simulink subsystem "F16_Quaternion"  (R2023b)
settings: Solver=VariableStepAuto  StartTime=0.0  StopTime=10.0  RelTol=1e-3
undefined symbols (not defined in the file): controlDeflections, dataBase, deltaLEF, e0_0, e1_0, e2_0, e3_0, pm_0, statesFinal, Vm_0, xme_0
libraries: sharedtransform x4, aerolibtransform2 x2, matrix_library x2, shared6dof x1
(part 1 of 2)
settings Model: Creator=cyber  LastModifiedBy=cyber

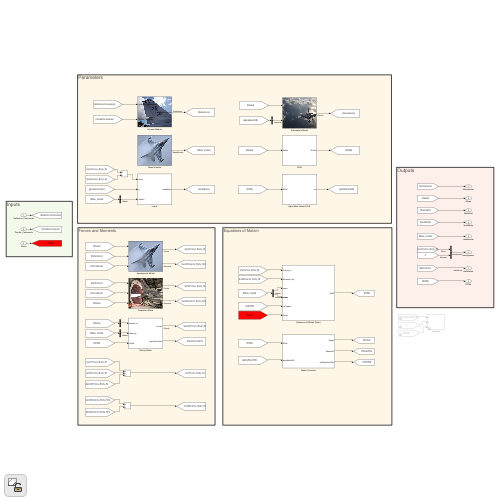
[thumbnail: Simulink's stored preview of the top-level diagram]
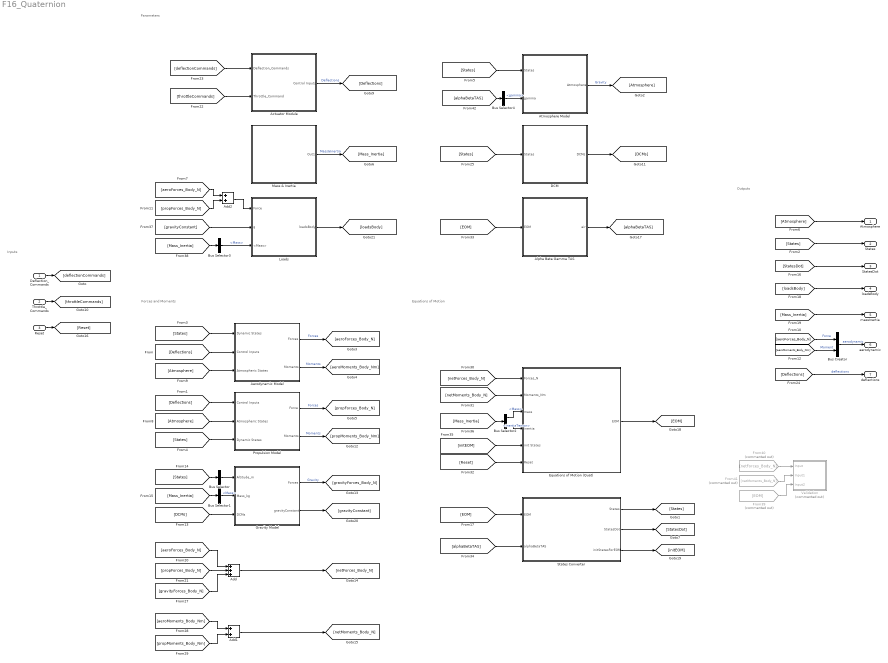
== system F16_Quaternion ==
  note: Forces and Moments
  note: Outputs
  note: Inputs
  note: Parameters
  note: Equations of Motion
  Deflection_Commands : Inport
  Throttle_Commands : Inport  Port=2
  Reset : Inport  Port=3
  Actuator Module : Subsystem
      mask Display: image('F16_ControlSurface.png'); % Use "Edit Image" on toolstrip to change.
  Add : Sum  Inputs=+++
  Add1 : Sum
  Add2 : Sum
  Aerodynamic Model : Subsystem
      mask Display: image('F16.PNG'); % Use "Edit Image" on toolstrip to change.
  "Alpha Beta Gamma TAS " : Subsystem
  Atmosphere Model : Subsystem
      mask Display: image('f16_atm.jpg'); % Use "Edit Image" on toolstrip to change.
  Bus Creator : BusCreator  Inputs=2
  Bus Selector : BusSelector  OutputSignals=Altitude  OutputAsBus=on
  Bus Selector1 : BusSelector  OutputSignals=Mass
  Bus Selector2 : BusSelector  OutputSignals=Mass,inertiaTensor
  Bus Selector3 : BusSelector  OutputSignals=Mass
  Bus Selector4 : BusSelector  OutputSignals=gamma
  DCM : Subsystem
  Equations of Motion (Quat) : Subsystem
  From39 : From  Commented=on  GotoTag=EOM
  From40 : From  Commented=on  GotoTag=netForces_Body_N
  From41 : From  Commented=on  GotoTag=netMoments_Body_N
  "Gravity Model " : Subsystem
  Loads : Subsystem
  Mass & Inertia : Subsystem
      mask Display: image('F16.PNG'); % Use "Edit Image" on toolstrip to change.
  Propulsion Model : Subsystem
      mask Display: image('F16_Engine.PNG'); % Use "Edit Image" on toolstrip to change.
  States Converter : Subsystem
  Validation : Subsystem  Commented=on
  Atmosphere : Outport
  States : Outport  Port=2
  StatesDot : Outport  Port=3
  loadsBody : Outport  Port=4
  massInertia : Outport  Port=5
  aerodynamic : Outport  Port=6
  deflections : Outport  Port=7
  wires:
  DCM/1(DCMs) -> [DCMs]
  [States] -> DCM/1(States)
  [Deflections] -> deflections/1  "deflections"
  Throttle_Commands/1 -> [throttleCommands]
  [deflectionCommands] -> Actuator Module/1(Deflection_Commands)
  Actuator Module/1(Control Inputs) -> [Deflections]  "Deflections"
  [throttleCommands] -> Actuator Module/2(Throttle_Command)
  Bus Creator/1 -> aerodynamic/1  "aerodynamic"
  [aeroMoments_Body_Nm] -> Bus Creator/2  "Moment"
  [aeroForces_Body_N] -> Bus Creator/1  "Force"
  [Mass_Inertia] -> massInertia/1
  [loadsBody] -> loadsBody/1
  [StatesDot] -> StatesDot/1
  [Atmosphere] -> Aerodynamic Model/3(Atmospheric States)
  [Atmosphere] -> Propulsion Model/2(Atmospheric States)
  [Atmosphere] -> Atmosphere/1
  [States] -> Atmosphere Model/1(States)
  [States] -> Propulsion Model/3(Dynamic States)
  [States] -> Aerodynamic Model/1(Dynamic States)
  [States] -> States/1
  [Deflections] -> Propulsion Model/1(Control Inputs)
  Deflection_Commands/1 -> [deflectionCommands]
  States Converter/2(StatesDot) -> [StatesDot]
  Atmosphere Model/1(Atmosphere) -> [Atmosphere]  "Gravity"
  [Deflections] -> Aerodynamic Model/2(Control Inputs)
  Aerodynamic Model/1(Forces) -> [aeroForces_Body_N]  "Forces"
  Aerodynamic Model/2(Moments) -> [aeroMoments_Body_Nm]  "Moments"
  States Converter/1(States) -> [States]
  Mass & Inertia/1(Out1) -> [Mass_Inertia]  "Mass&Inertia"
  Propulsion Model/2(Moments) -> [propMoments_Body_Nm]  "Moments"
  Propulsion Model/1(Force) -> [propForces_Body_N]  "Forces"
  [DCMs] -> "Gravity Model "/3(DCMs)
  [States] -> Bus Selector/1
  Bus Selector/1 -> "Gravity Model "/1(Altitude_m)
  [Mass_Inertia] -> Bus Selector1/1
  Bus Selector1/1 -> "Gravity Model "/2(Mass_kg)  "<Mass>"
  "Gravity Model "/1(Forces) -> [gravityForces_Body_N]  "Gravity"
  [propForces_Body_N] -> Add/2
  [aeroForces_Body_N] -> Add/1
  [gravityForces_Body_N] -> Add/3
  Add/1 -> [netForces_Body_N]
  [aeroMoments_Body_Nm] -> Add1/1
  [propMoments_Body_Nm] -> Add1/2
  Add1/1 -> [netMoments_Body_N]
  [netForces_Body_N] -> Equations of Motion (Quat)/1(Forces_N)
  [netMoments_Body_N] -> Equations of Motion (Quat)/2(Moments_Nm)
  Reset/1 -> [Reset]
  [Reset] -> Equations of Motion (Quat)/6(Reset)
  "Alpha Beta Gamma TAS "/1(air) -> [alphaBetaTAS]
  Equations of Motion (Quat)/1(EOM) -> [EOM]
  [EOM] -> "Alpha Beta Gamma TAS "/1(EOM)
  [EOM] -> States Converter/1(EOM)
  [alphaBetaTAS] -> States Converter/2(alphaBetaTAS)
  States Converter/3(initStatesForEOM) -> [initEOM]
  [initEOM] -> Equations of Motion (Quat)/5(init States)
  [Mass_Inertia] -> Bus Selector2/1
  Bus Selector2/1 -> Equations of Motion (Quat)/3(mass)  "<Mass>"
  Bus Selector2/2 -> Equations of Motion (Quat)/4(inertia)  "<inertiaTensor>"
  "Gravity Model "/2(gravityConstant) -> [gravityConstant]
  Bus Selector3/1 -> Loads/3(<Mass>)  "<Mass>"
  [aeroForces_Body_N] -> Add2/1
  [propForces_Body_N] -> Add2/2
  Add2/1 -> Loads/1(Force)
  [gravityConstant] -> Loads/2(g)
  [Mass_Inertia] -> Bus Selector3/1
  Loads/1(loadsBody) -> [loadsBody]
  From39/1 -> Validation/3(Input2)
  From41/1 -> Validation/2(Input1)
  From40/1 -> Validation/1(Input)
  [alphaBetaTAS] -> Bus Selector4/1
  Bus Selector4/1 -> Atmosphere Model/2(gamma)  "<gamma>"

== system F16_Quaternion/Actuator Module ==
  Deflection_Commands : Inport
  Throttle_Command : Inport  Port=2
  Bus Creator : BusCreator  Inputs=6
  Demux : Demux  Outputs=6
  First Order Aileron Actuator : Subsystem
  First Order HT Actuator : Subsystem
  First Order Rudder Actuator : Subsystem
  First Order Throttle Actuator : Subsystem
  Leading Edge Flap : Constant  Value=deltaLEF
  Speed Brake : Constant  Value=0
  Terminator : Terminator
  Terminator1 : Terminator
  Terminator2 : Terminator
  Control Inputs : Outport
  wires:
  Bus Creator/1 -> Control Inputs/1
  First Order Throttle Actuator/1(Output) -> Bus Creator/4  "Throttle"
  Speed Brake/1 -> Bus Creator/6  "Speed Brake"
  Demux/1 -> [HorizontalTail]
  Demux/2 -> [Aileron]
  Demux/3 -> [Rudder]
  Demux/4 -> Terminator/1
  Demux/5 -> Terminator2/1
  Demux/6 -> Terminator1/1
  Deflection_Commands/1 -> Demux/1
  Leading Edge Flap/1 -> Bus Creator/5  "LEF"
  [HorizontalTail] -> First Order HT Actuator/1(Deflection)  "Horizontal Tail Command"
  [Aileron] -> First Order Aileron Actuator/1(Deflection)  "Aileron Command"
  [Rudder] -> First Order Rudder Actuator/1(Deflection)  "Rudder Command"
  First Order HT Actuator/1(Output) -> Bus Creator/1  "Horizontal Tail"
  First Order Aileron Actuator/1(Output) -> Bus Creator/2  "Aileron"
  First Order Rudder Actuator/1(Output) -> Bus Creator/3  "Rudder"
  Throttle_Command/1 -> [Throttle_Command]
  [Throttle_Command] -> First Order Throttle Actuator/1(Deflection)  "Throttle Command"

== system F16_Quaternion/Aerodynamic Model ==
  Dynamic States : Inport
  Control Inputs : Inport  Port=2
  Atmospheric States : Inport  Port=3
  Bus Creator : BusCreator  Inputs=2
  Bus Selector : BusSelector  OutputSignals=Dynamic Pressure
  Constant : Constant  Value=dataBase.Sw
  Demux1 : Demux  Outputs=3
  Force Coeffs : Subsystem
  Gain : Gain  Gain=dataBase.MAC*dataBase.Sw
  Gain1 : Gain  Gain=dataBase.b*dataBase.Sw
  Gain2 : Gain  Gain=dataBase.b*dataBase.Sw
  Moment Coeffs : Subsystem
  Mux : Mux  Inputs=3
  Mux1 : Mux  Inputs=3
  Mux2 : Mux  Inputs=3
  Product : Product  Inputs=3
  Product1 : Product
  Product2 : Product
  Product3 : Product
  Selector : Selector  InputPortWidth=3  IndexOptions=Index vector (dialog)  Indices=[2,1,3]  OutputSizes=1
  Forces : Outport
  Moments : Outport  Port=2
  wires:
  Selector/1 -> Moments/1
  Force Coeffs/3(" CZ") -> Bus Creator/2, Mux/3  "CZ"
  Force Coeffs/2(" CY") -> Bus Creator/1, Mux/2  "CY"
  Force Coeffs/1(" CX") -> Mux/1
  Mux/1 -> Product/2
  Moment Coeffs/1(" Cm") -> Mux1/1
  Mux1/1 -> Demux1/1
  Moment Coeffs/3(" Cn") -> Mux1/3
  Moment Coeffs/2(" Cl") -> Mux1/2
  Bus Creator/1 -> Moment Coeffs/1(Force Effects on Moments)
  Dynamic States/1 -> Moment Coeffs/2(Dynamic States), Force Coeffs/1(Dynamic States)
  Control Inputs/1 -> Moment Coeffs/3(Control Inputs), Force Coeffs/2(Control Inputs)
  Atmospheric States/1 -> Bus Selector/1
  Bus Selector/1 -> [DynamicPressure]  "<Dynamic Pressure>"
  [DynamicPressure] -> Product/1
  Constant/1 -> Product/3
  Product/1 -> Forces/1
  Demux1/1 -> Gain/1
  Gain/1 -> Product1/2
  [DynamicPressure] -> Product2/1, Product3/1, Product1/1
  Demux1/2 -> Gain1/1
  Demux1/3 -> Gain2/1
  Gain1/1 -> Product2/2
  Gain2/1 -> Product3/2
  Product3/1 -> Mux2/3
  Product2/1 -> Mux2/2
  Product1/1 -> Mux2/1
  Mux2/1 -> Selector/1

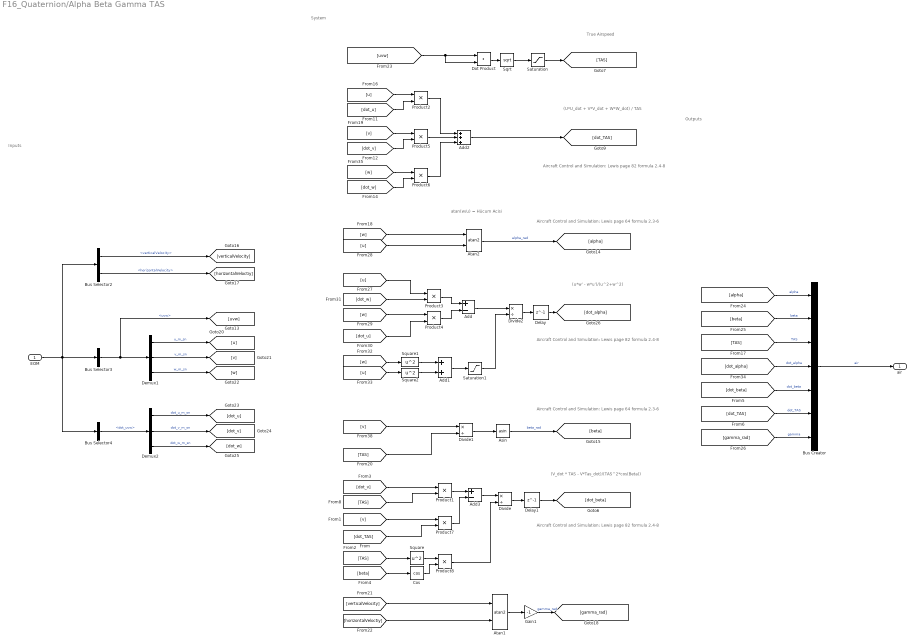
== system F16_Quaternion/Alpha Beta Gamma TAS  ==
  note: Aircraft Control and Simulation: Lewis page 64 formula 2.3-6
  note: Aircraft Control and Simulation: Lewis page 64 formula 2.3-6
  note: Aircraft Control and Simulation: Lewis page 82 formula 2.4-8
  note: Aircraft Control and Simulation: Lewis page 82 formula 2.4-8
  note: System
  note: Outputs
  note: Inputs
  note: (u*w' - w*u')/(u^2+w^2)
  note: atan(w/u) = Hücum Acisi
  note: Aircraft Control and Simulation: Lewis page 82 formula 2.4-8
  note: (U*U_dot + V*V_dot + W*W_dot) / TAS
  note: (V_dot * TAS - V*Tas_dot)/(TAS^2*cos(Beta))
  note: True Airspeed
  EOM : Inport  OutDataTypeStr=double
  Add : Sum  Inputs=+-
  Add1 : Sum
  Add2 : Sum  Inputs=3
  Add3 : Sum  Inputs=+-
  Asin : Trigonometry  Operator=asin
  Atan1 : Trigonometry  Operator=atan2
  Atan2 : Trigonometry  Operator=atan2
  Bus Creator : BusCreator  Inputs=7
  Bus Selector2 : BusSelector  OutputSignals=verticalVelocity,horizontalVelocity
  Bus Selector3 : BusSelector  OutputSignals=uvw
  Bus Selector4 : BusSelector  OutputSignals=dot_uvw
  Cos : Trigonometry  Operator=cos
  Delay : Delay  DelayLength=1  InitialCondition=0
  Delay1 : Delay  DelayLength=1
  Demux1 : Demux  Outputs=3
  Demux2 : Demux  Outputs=3
  Divide : Product  Inputs=*/
  Divide1 : Product  Inputs=*/
  Divide2 : Product  Inputs=*/
  Dot Product : DotProduct  OutDataTypeStr=Inherit: Inherit via internal rule
  Gain1 : Gain  Gain=-1
  Product{1..8} (8 alike) : Product
  Saturation : Saturate  UpperLimit=inf  LowerLimit=0.000000001
  Saturation1 : Saturate  UpperLimit=inf  LowerLimit=0.000000001
  Sqrt : Sqrt
  Square : Math  Operator=square
  Square1 : Math  Operator=square
  Square2 : Math  Operator=square
  air : Outport
  wires:
  [gamma_rad] -> Bus Creator/7  "gamma"
  [dot_TAS] -> Bus Creator/6  "dot_TAS"
  [dot_beta] -> Bus Creator/5  "dot_beta"
  [dot_alpha] -> Bus Creator/4  "dot_alpha"
  [alpha] -> Bus Creator/1  "alpha"
  [TAS] -> Bus Creator/3  "TAS"
  [beta] -> Bus Creator/2  "beta"
  Divide/1 -> Delay1/1
  Product8/1 -> Divide/2
  Cos/1 -> Product8/2
  Square/1 -> Product8/1
  [beta] -> Cos/1
  Add3/1 -> Divide/1
  [TAS] -> Square/1
  [v] -> Product7/1
  [dot_TAS] -> Product7/2
  Product7/1 -> Add3/2
  Product1/1 -> Add3/1
  [TAS] -> Product1/2
  [dot_v] -> Product1/1
  Delay1/1 -> [dot_beta]
  Add2/1 -> [dot_TAS]
  Product2/1 -> Add2/1
  Product6/1 -> Add2/3
  Product5/1 -> Add2/2
  [dot_w] -> Product6/2
  [w] -> Product6/1
  [v] -> Product5/1
  [dot_v] -> Product5/2
  [dot_u] -> Product2/2
  [u] -> Product2/1
  Delay/1 -> [dot_alpha]
  Saturation1/1 -> Divide2/2
  Saturation/1 -> [TAS]
  Divide2/1 -> Delay/1
  Add1/1 -> Saturation1/1
  Square2/1 -> Add1/2
  Square1/1 -> Add1/1
  [u] -> Square2/1
  [w] -> Square1/1
  Add/1 -> Divide2/1
  Product4/1 -> Add/2
  Product3/1 -> Add/1
  [dot_u] -> Product4/2
  [w] -> Product4/1
  [dot_w] -> Product3/2
  [u] -> Product3/1
  Bus Selector4/1 -> Demux2/1  "<dot_uvw>"
  Demux2/1 -> [dot_u]  "dot_u_m_sn"
  Demux2/2 -> [dot_v]  "dot_v_m_sn"
  Demux2/3 -> [dot_w]  "dot_w_m_sn"
  Demux1/3 -> [w]  "w_m_sn"
  Demux1/2 -> [v]  "v_m_sn"
  Demux1/1 -> [u]  "u_m_sn"
  [uvw] -> Dot Product/1, Dot Product/2
  Sqrt/1 -> Saturation/1
  Dot Product/1 -> Sqrt/1
  Gain1/1 -> [gamma_rad]  "gamma_rad"
  Atan1/1 -> Gain1/1
  [horizontalVeloctiy] -> Atan1/2
  [verticalVelocity] -> Atan1/1
  Bus Selector2/2 -> [horizontalVeloctiy]  "<horizontalVelocity>"
  Bus Selector2/1 -> [verticalVelocity]  "<verticalVelocity>"
  Asin/1 -> [beta]  "beta_rad"
  Divide1/1 -> Asin/1
  [TAS] -> Divide1/2
  [v] -> Divide1/1
  Atan2/1 -> [alpha]  "alpha_rad"
  [w] -> Atan2/1
  [u] -> Atan2/2
  Bus Selector3/1 -> Demux1/1, [uvw]  "<uvw>"
  EOM/1 -> Bus Selector3/1, Bus Selector2/1, Bus Selector4/1
  Bus Creator/1 -> air/1  "air"

== system F16_Quaternion/Atmosphere Model ==
  States : Inport
  gamma : Inport  Port=2
  Bus Creator : BusCreator  Inputs=8
  Bus Selector : BusSelector  OutputSignals=Altitude,Velocity
  MATLAB Function : MATLAB Function  TreatAsAtomicUnit=on
  Atmosphere : Outport
  wires:
  MATLAB Function/7(speedOfSound) -> Bus Creator/7  "speedOfSound"
  gamma/1 -> Bus Creator/8  "gamma"
  States/1 -> Bus Selector/1
  MATLAB Function/2(T) -> Bus Creator/2  "Temperature"
  MATLAB Function/3(P) -> Bus Creator/3  "Pressure"
  MATLAB Function/4(rho) -> Bus Creator/4  "Density"
  MATLAB Function/5(Qdyn) -> Bus Creator/5  "Dynamic Pressure"
  MATLAB Function/6(M) -> Bus Creator/6  "Mach"
  MATLAB Function/1(g) -> Bus Creator/1  "Gravity"
  Bus Creator/1 -> Atmosphere/1
  Bus Selector/1 -> MATLAB Function/1(h)  "<Altitude>"
  Bus Selector/2 -> MATLAB Function/2(V)  "<Velocity>"

== system F16_Quaternion/DCM ==
  note: Body to Wind
  note: Body to Stability
  note: Earth to Body
  States : Inport
  Bus Creator : BusCreator  Inputs=3
  Bus Selector : BusSelector  OutputSignals=Phi,Theta,Psi,Alpha,Beta
  Constant1 : Constant  Value=0
  Direction Cosine Matrix Body to Wind1 : aerolibtransform2/Direction Cosine Matrix Body to Wind
  Direction Cosine Matrix Body to Wind2 : aerolibtransform2/Direction Cosine Matrix Body to Wind
  Mux : Mux  Inputs=3
  Mux1 : Mux  Inputs=2
  Mux3 : Mux  Inputs=2
  Rotation Angles to Direction Cosine Matrix : sharedtransform/Rotation Angles to Direction Cosine Matrix  rotationOrder=ZYX  aMode=aMode
  DCMs : Outport
  wires:
  Bus Selector/5 -> [beta]  "<Beta>"
  [beta] -> Mux1/2  "beta_rad"
  Mux1/1 -> Direction Cosine Matrix Body to Wind2/1
  [alpha] -> Mux1/1
  Direction Cosine Matrix Body to Wind2/1 -> Bus Creator/3  "DCMwb"
  Bus Selector/4 -> [alpha]  "<Alpha>"
  Direction Cosine Matrix Body to Wind1/1 -> Bus Creator/2  "DCMsb"
  [alpha] -> Mux3/1
  Mux3/1 -> Direction Cosine Matrix Body to Wind1/1
  Constant1/1 -> Mux3/2  "beta_rad"
  Mux/1 -> Rotation Angles to Direction Cosine Matrix/1
  States/1 -> Bus Selector/1
  Bus Selector/1 -> [phi]  "<Phi>"
  Bus Selector/2 -> [theta]  "<Theta>"
  Bus Selector/3 -> [psi]  "<Psi>"
  [theta] -> Mux/2
  [phi] -> Mux/3
  [psi] -> Mux/1
  Rotation Angles to Direction Cosine Matrix/1 -> Bus Creator/1  "DCMbe"
  Bus Creator/1 -> DCMs/1

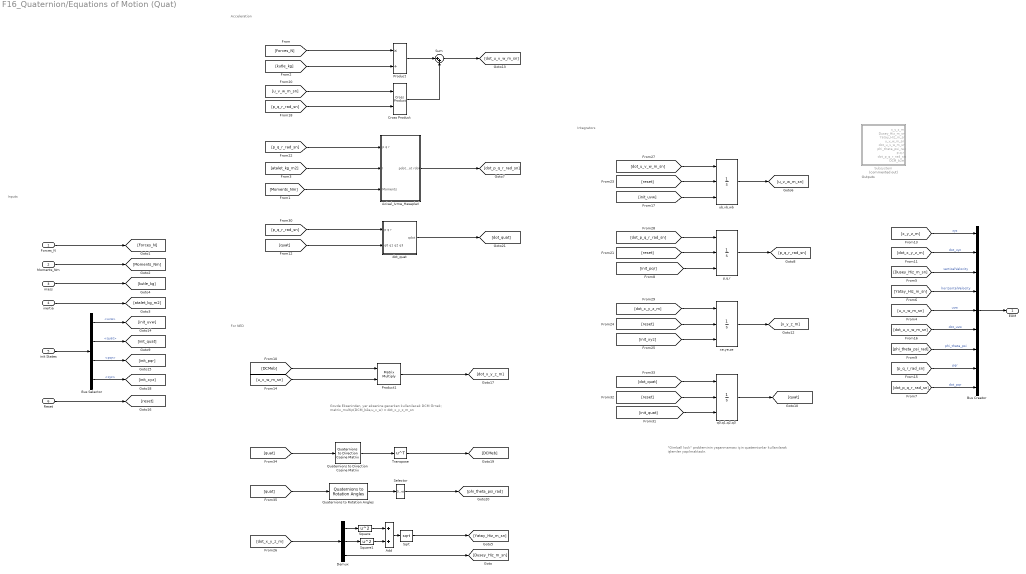
== system F16_Quaternion/Equations of Motion (Quat) ==
  note: "Gimball lock" probleminin yaşanmaması için quaternionlar kullanılarak işlemler yapılmaktadır.
  note: Acceleration
  note: For NED
  note: Inputs
  note: Outputs
  note: Integrators
  note: Govde Ekseninden, yer eksenine gecerken kullanilacak DCM
      |
      | Örnek;
      | matrix_multip(DCM_b2e,u_v_w) = dot_x_y_z_m_sn
  Forces_N : Inport  OutDataTypeStr=double
  Moments_Nm : Inport  Port=2  OutDataTypeStr=double
  mass : Inport  Port=3
  inertia : Inport  Port=4
  init States : Inport  Port=5
  Reset : Inport  Port=6
  Acisal_Ivme_Hesaplari : Subsystem
  Add : Sum
  Bus Creator : BusCreator  Inputs=9
  Bus Selector : BusSelector  OutputSignals=uvw,quat,pqr,xyz
  Cross Product : matrix_library/Cross Product
  Demux : Demux  Outputs=3
  Product : Product  Inputs=*/  SaturateOnIntegerOverflow=on  OutDataTypeStr=Inherit: Same as first input
  Product1 : Product  Multiplication=Matrix(*)
  Quaternions to Direction Cosine Matrix : sharedtransform/Quaternions to  Direction Cosine Matrix  aMode=aMode
  Quaternions to Rotation Angles : sharedtransform/Quaternions to Rotation Angles  rotationOrder=ZYX  aMode=aMode
  Selector : Selector  InputPortWidth=3  IndexOptions=Index vector (dialog)  Indices=[3 2 1]  OutputSizes=1
  Sqrt : Sqrt
  Square : Math  Operator=square
  Square1 : Math  Operator=square
  Subsystem : Subsystem  Commented=on
  Sum : Sum  Inputs=|++  SaturateOnIntegerOverflow=on
  Transpose : Math  Operator=transpose  SignedPower=on
  dot_quat : Subsystem
  "p,q,r " : Integrator  ExternalReset=rising  InitialConditionSource=external  InitialCondition=pm_0
  q0,q1,q2,q3 : Integrator  ExternalReset=rising  InitialConditionSource=external  InitialCondition=[e0_0 e1_0 e2_0 e3_0]
  ub,vb,wb : Integrator  ExternalReset=rising  InitialConditionSource=external  InitialCondition=Vm_0
  xe,ye,ze : Integrator  ExternalReset=rising  InitialConditionSource=external  InitialCondition=xme_0
  EOM : Outport
  wires:
  inertia/1 -> [atalet_kg_m2]
  mass/1 -> [kutle_kg]
  Bus Selector/2 -> [init_quat]  "<quat>"
  init States/1 -> Bus Selector/1
  [dot_x_y_z_m] -> Bus Creator/2  "dot_xyz"
  Bus Creator/1 -> EOM/1
  [u_v_w_m_sn] -> Product1/2
  [dot_p_q_r_rad_sn] -> Bus Creator/9  "dot_pqr"
  [p_q_r_rad_sn] -> Bus Creator/8  "pqr"
  [phi_theta_psi_rad] -> Bus Creator/7  "phi_theta_psi"
  [dot_u_v_w_m_sn] -> Bus Creator/6  "dot_uvw"
  [u_v_w_m_sn] -> Bus Creator/5  "uvw"
  [Yatay_Hiz_m_sn] -> Bus Creator/4  "horizontalVelocity"
  [Dusey_Hiz_m_sn] -> Bus Creator/3  "verticalVelocity"
  [x_y_z_m] -> Bus Creator/1  "xyz"
  [reset] -> q0,q1,q2,q3/2
  [reset] -> xe,ye,ze/2
  [reset] -> "p,q,r "/2
  [reset] -> ub,vb,wb/2
  [quat] -> Quaternions to Rotation Angles/1
  [quat] -> Quaternions to Direction Cosine Matrix/1
  dot_quat/1(qdot) -> [dot_quat]
  [p_q_r_rad_sn] -> dot_quat/1(p q r)
  [quat] -> dot_quat/2(q0 q1 q2 q3)
  [init_quat] -> q0,q1,q2,q3/3
  [dot_quat] -> q0,q1,q2,q3/1
  Selector/1 -> [phi_theta_psi_rad]
  q0,q1,q2,q3/1 -> [quat]
  Quaternions to Direction Cosine Matrix/1 -> Transpose/1
  Quaternions to Rotation Angles/1 -> Selector/1
  Transpose/1 -> [DCMeb]
  [DCMeb] -> Product1/1
  [dot_x_y_z_m] -> xe,ye,ze/1
  [dot_p_q_r_rad_sn] -> "p,q,r "/1
  [dot_u_v_w_m_sn] -> ub,vb,wb/1
  [dot_x_y_z_m] -> Demux/1
  [init_xyz] -> xe,ye,ze/3
  Bus Selector/4 -> [init_xyz]  "<xyz>"
  [p_q_r_rad_sn] -> Acisal_Ivme_Hesaplari/1(p q r)
  Reset/1 -> [reset]
  [u_v_w_m_sn] -> Cross Product/1
  [init_pqr] -> "p,q,r "/3
  Bus Selector/3 -> [init_pqr]  "<pqr>"
  [p_q_r_rad_sn] -> Cross Product/2
  Bus Selector/1 -> [init_uvw]  "<uvw>"
  [init_uvw] -> ub,vb,wb/3
  xe,ye,ze/1 -> [x_y_z_m]
  Sqrt/1 -> [Yatay_Hiz_m_sn]
  Add/1 -> Sqrt/1
  Square1/1 -> Add/2
  Square/1 -> Add/1
  Demux/3 -> [Dusey_Hiz_m_sn]
  Demux/2 -> Square1/1
  Demux/1 -> Square/1
  Moments_Nm/1 -> [Moments_Nm]
  Forces_N/1 -> [Forces_N]
  [atalet_kg_m2] -> Acisal_Ivme_Hesaplari/2(I)
  Product1/1 -> [dot_x_y_z_m]
  Cross Product/1 -> Sum/2
  [Moments_Nm] -> Acisal_Ivme_Hesaplari/3(Moments)
  Product/1 -> Sum/1
  [kutle_kg] -> Product/2
  Acisal_Ivme_Hesaplari/1(pdot qdot rdot) -> [dot_p_q_r_rad_sn]
  [Forces_N] -> Product/1
  "p,q,r "/1 -> [p_q_r_rad_sn]
  Sum/1 -> [dot_u_v_w_m_sn]
  ub,vb,wb/1 -> [u_v_w_m_sn]

== system F16_Quaternion/Gravity Model  ==
  note: Earth to Body DCM
  note: g = 9.80665*(6371020/(6371020+h))^2;
      | Calculation will change in further release
  Altitude_m : Inport
  Mass_kg : Inport  Port=2
  DCMs : Inport  Port=3
  Add : Sum
  Bus Selector : BusSelector  OutputSignals=DCMbe
  Constant : Constant  Value=9.80665
  Constant1 : Constant  Value=6371020
  Constant2 : Constant  Value=6371020
  Constant3 : Constant  Value=[0,0]
  Divide : Product  Inputs=*/
  Divide1 : Product  Inputs=**
  MatrixMultiply : Product  Multiplication=Matrix(*)
  Mux : Mux  Inputs=2
  Product : Product
  Square : Math  Operator=square
  Forces : Outport
  gravityConstant : Outport  Port=2
  wires:
  [g] -> gravityConstant/1
  MatrixMultiply/1 -> Forces/1
  [DCMbe] -> MatrixMultiply/1
  [gravityForce_NED_N] -> MatrixMultiply/2
  Mux/1 -> [gravityForce_NED_N]
  Constant3/1 -> Mux/1
  Product/1 -> Mux/2
  Divide1/1 -> Product/1, [g]
  Mass_kg/1 -> Product/2
  Square/1 -> Divide1/2
  Constant/1 -> Divide1/1
  Divide/1 -> Square/1
  Add/1 -> Divide/2
  Constant1/1 -> Divide/1
  Altitude_m/1 -> Add/2
  Constant2/1 -> Add/1
  Bus Selector/1 -> [DCMbe]  "<DCMbe>"
  DCMs/1 -> Bus Selector/1

== system F16_Quaternion/Loads ==
  Force : Inport
  g : Inport  Port=2
  <Mass> : Inport  Port=3
  Bus Creator : BusCreator  Inputs=3
  Demux : Demux  Outputs=3
  Divide : Product  Inputs=*/
  Gain : Gain  Gain=[1,1,-1]
  Product : Product
  loadsBody : Outport
  wires:
  Divide/1 -> Demux/1
  Product/1 -> Divide/2
  Gain/1 -> Divide/1
  Demux/3 -> Bus Creator/3  "Nz"
  Bus Creator/1 -> loadsBody/1
  Demux/1 -> Bus Creator/1  "Nx"
  Demux/2 -> Bus Creator/2  "Ny"
  <Mass>/1 -> Product/2
  g/1 -> Product/1
  Force/1 -> Gain/1

== system F16_Quaternion/Mass & Inertia ==
  Bus Creator : BusCreator  Inputs=2
  MATLAB Function : MATLAB Function  TreatAsAtomicUnit=on
  Out1 : Outport
  wires:
  MATLAB Function/1(Mass) -> Bus Creator/1
  MATLAB Function/2(inertiaTensor) -> Bus Creator/2
  Bus Creator/1 -> Out1/1

== system F16_Quaternion/Propulsion Model ==
  Control Inputs : Inport
  Atmospheric States : Inport  Port=2
  Dynamic States : Inport  Port=3
  Bus Selector3 : BusSelector  OutputSignals=Throttle
  Bus Selector4 : BusSelector  OutputSignals=Mach
  Bus Selector5 : BusSelector  OutputSignals=Altitude,Q,R
  Constant : Constant  Value=[0,0]
  Gain1 : Gain  Gain=4.4882
  Gain2 : Gain  Gain=4.4882
  Gain3 : Gain  Gain=4.4882
  Idle : Lookup_n-D  BreakpointsForDimension1=dataBase.Engine.f16_EngineData.BP.idle.mach  BreakpointsForDimension2=dataBase.Engine.f16_EngineData.BP.idle.alt_ft  Table=dataBase.Engine.f16_EngineData.data.Thrust_lbs.idle  ExtrapMethod=Clip  InternalRulePriority=Speed  RndMeth=Simplest
      settings: InputPortMap=u0,u1
  MATLAB Function : MATLAB Function  TreatAsAtomicUnit=on
  MATLAB Function1 : MATLAB Function  TreatAsAtomicUnit=on
  Maximum : Lookup_n-D  BreakpointsForDimension1=dataBase.Engine.f16_EngineData.BP.max.mach  BreakpointsForDimension2=dataBase.Engine.f16_EngineData.BP.max.alt_ft  Table=dataBase.Engine.f16_EngineData.data.Thrust_lbs.max  ExtrapMethod=Clip  InternalRulePriority=Speed  RndMeth=Simplest
      settings: InputPortMap=u0,u1
  Military : Lookup_n-D  BreakpointsForDimension1=dataBase.Engine.f16_EngineData.BP.mil.mach  BreakpointsForDimension2=dataBase.Engine.f16_EngineData.BP.mil.alt_ft  Table=dataBase.Engine.f16_EngineData.data.Thrust_lbs.mil  ExtrapMethod=Clip  InternalRulePriority=Speed  RndMeth=Simplest
      settings: InputPortMap=u0,u1
  Mux : Mux  Inputs=2
  m2ft : Gain  Gain=1/0.3048
  Force : Outport
  Moments : Outport  Port=2
  wires:
  MATLAB Function/1(T_moment) -> Moments/1
  Constant/1 -> Mux/2
  Mux/1 -> Force/1
  MATLAB Function1/1(Thrust) -> Mux/1
  [Tidle] -> MATLAB Function1/1(Tidle)
  [Tmil] -> MATLAB Function1/2(Tmil)
  Gain3/1 -> [Tmax]
  Idle/1 -> Gain1/1
  Gain1/1 -> [Tidle]
  Maximum/1 -> Gain3/1
  Military/1 -> Gain2/1
  [Tmax] -> MATLAB Function1/3(Tmax)
  m2ft/1 -> Maximum/2, Military/2, Idle/2
  Gain2/1 -> [Tmil]
  Control Inputs/1 -> Bus Selector3/1
  Bus Selector3/1 -> MATLAB Function1/4(Throttle)  "<Throttle>"
  Bus Selector4/1 -> Maximum/1, Military/1, Idle/1  "<Mach>"
  Bus Selector5/1 -> m2ft/1  "<Altitude>"
  Dynamic States/1 -> Bus Selector5/1
  Atmospheric States/1 -> Bus Selector4/1
  Bus Selector5/2 -> [Q]  "<Q>"
  Bus Selector5/3 -> [R]  "<R>"
  [Q] -> MATLAB Function/1(Q)
  [R] -> MATLAB Function/2(R)

== system F16_Quaternion/States Converter ==
  note: Not used. So not critical.
  EOM : Inport
  alphaBetaTAS : Inport  Port=2
  Bus Creator2 : BusCreator  Inputs=12
  Bus Creator3 : BusCreator  Inputs=12
  Bus Selector : BusSelector  OutputSignals=alpha,beta,TAS,dot_alpha,dot_beta,dot_TAS,gamma
  Bus Selector1 : BusSelector  OutputSignals=xyz,dot_xyz,phi_theta_psi,pqr,dot_pqr
  Constant : Constant  Value=statesFinal
  Demux{,4..8} (6 alike) : Demux  Outputs=3
  Derivative : Derivative
  Gain : Gain  Gain=-1
  Gain1 : Gain  Gain=-1
  States Converter : Subsystem
  Terminator : Terminator
  States : Outport
  StatesDot : Outport  Port=2
  initStatesForEOM : Outport  Port=3
  wires:
  States Converter/1(EOM) -> initStatesForEOM/1
  Constant/1 -> States Converter/1(States)
  Gain1/1 -> Bus Creator3/12  "AltitudeDot"
  [dot_xyz] -> Demux8/1
  Derivative/1 -> Demux7/1
  [phi_theta_psi] -> Derivative/1
  [dot_pqr] -> Demux6/1
  Bus Selector1/2 -> [dot_xyz]  "<dot_xyz>"
  [pqr] -> Demux5/1
  Demux4/1 -> Bus Creator2/3  "Phi"
  [phi_theta_psi] -> Demux4/1
  Gain/1 -> Bus Creator2/12  "Altitude"
  [xyz] -> Demux/1
  Bus Selector1/5 -> [dot_pqr]  "<dot_pqr>"
  Bus Selector1/4 -> [pqr]  "<pqr>"
  Bus Selector1/3 -> [phi_theta_psi]  "<phi_theta_psi>"
  Bus Selector1/1 -> [xyz]  "<xyz>"
  Bus Selector/7 -> Terminator/1  "<gamma>"
  EOM/1 -> Bus Selector1/1
  Bus Selector/4 -> [dot_alpha]  "<dot_alpha>"
  Bus Selector/5 -> [dot_beta]  "<dot_beta>"
  Bus Selector/6 -> [dot_TAS]  "<dot_TAS>"
  Bus Selector/3 -> [TAS]  "<TAS>"
  Bus Selector/2 -> [beta]  "<beta>"
  Bus Selector/1 -> [alpha]  "<alpha>"
  alphaBetaTAS/1 -> Bus Selector/1
  [alpha] -> Bus Creator2/1  "Alpha"
  Demux8/1 -> Bus Creator3/10  "NorthDot"
  Demux4/3 -> Bus Creator2/5  "Psi"
  Demux7/3 -> Bus Creator3/5  "PsiDot"
  Demux/2 -> Bus Creator2/11  "East"
  Demux7/1 -> Bus Creator3/3  "PhiDot"
  Bus Creator2/1 -> States/1
  [dot_beta] -> Bus Creator3/2  "BetaDot"
  Demux8/3 -> Gain1/1
  Demux6/1 -> Bus Creator3/6  "PDot"
  [beta] -> Bus Creator2/2  "Beta"
  Demux6/3 -> Bus Creator3/8  "RDot"
  Demux8/2 -> Bus Creator3/11  "EastDot"
  Demux5/3 -> Bus Creator2/8  "R"
  [dot_alpha] -> Bus Creator3/1  "AlphaDot"
  Demux7/2 -> Bus Creator3/4  "ThetaDot"
  Demux4/2 -> Bus Creator2/4  "Theta"
  Demux/3 -> Gain/1
  Demux5/1 -> Bus Creator2/6  "P"
  Demux5/2 -> Bus Creator2/7  "Q"
  Bus Creator3/1 -> StatesDot/1
  [dot_TAS] -> Bus Creator3/9  "VelocityDot"
  Demux6/2 -> Bus Creator3/7  "QDot"
  Demux/1 -> Bus Creator2/10  "North"
  [TAS] -> Bus Creator2/9  "Velocity"

== system F16_Quaternion/Validation ==
  Input : Inport
  Input1 : Inport  Port=2
  Input2 : Inport  Port=3
  6DOF (Quaternion) : shared6dof/6DOF (Euler Angles)  units=Metric (MKS)  mtype=Fixed  rep=Quaternion  xme_0=init_xyz  Vm_0=init_uvw  eul_0=init_phi_theta_psi  pm_0=init_pqr  mass_0=Mass  mass_e=0.5  mass_f=2.0  inertia=inertiaTensor  inertia_e=eye(3)  inertia_f=2*eye(3)  k_quat=1.0  vre_flag=on  abi_flag=off  aMode=0  xme_statename=''  Vm_statename=''  eul_statename=''  quat_statename=''  pm_statename=''  mass_statename=''
      settings: LibrarySourceBlock=aerolib6dof2/6DOF (Quaternion)
  Add{3..8} (6 alike) : Sum  Inputs=+-
  Bus Selector1 : BusSelector  OutputSignals=xyz
  Bus Selector2 : BusSelector  OutputSignals=phi_theta_psi
  Bus Selector3 : BusSelector  OutputSignals=uvw
  Bus Selector4 : BusSelector  OutputSignals=dot_xyz
  Bus Selector5 : BusSelector  OutputSignals=pqr
  Bus Selector6 : BusSelector  OutputSignals=dot_pqr
  Scope : Scope  NumInputPorts=6
  Terminator : Terminator
  Terminator1 : Terminator
  wires:
  Bus Selector6/1 -> Add8/2  "<dot_pqr>"
  Bus Selector5/1 -> Add7/2  "<pqr>"
  Bus Selector3/1 -> Add6/2  "<uvw>"
  Bus Selector2/1 -> Add5/2  "<phi_theta_psi>"
  Bus Selector1/1 -> Add4/2  "<xyz>"
  [EOM] -> Bus Selector4/1, Bus Selector3/1, Bus Selector5/1, Bus Selector6/1, Bus Selector2/1, Bus Selector1/1
  Bus Selector4/1 -> Add3/2  "<dot_xyz>"
  Input2/1 -> [EOM]
  Input1/1 -> [netMoments_Body_N]
  Input/1 -> [netForces_Body_N]
  6DOF (Quaternion)/1 -> Add3/1
  6DOF (Quaternion)/2 -> Add4/1
  [netForces_Body_N] -> 6DOF (Quaternion)/1
  6DOF (Quaternion)/7 -> Add8/1
  6DOF (Quaternion)/5 -> Add6/1
  Add6/1 -> Scope/4
  [netMoments_Body_N] -> 6DOF (Quaternion)/2
  6DOF (Quaternion)/8 -> Terminator1/1
  6DOF (Quaternion)/4 -> Terminator/1
  Add4/1 -> Scope/2
  Add3/1 -> Scope/1
  Add5/1 -> Scope/3
  6DOF (Quaternion)/3 -> Add5/1
  Add7/1 -> Scope/5
  6DOF (Quaternion)/6 -> Add7/1
  Add8/1 -> Scope/6

== system F16_Quaternion/Actuator Module/First Order Aileron Actuator ==
  Deflection : Inport
  Gain : Gain  Gain=1/0.0495
  Integrator : Integrator  ExternalReset=either  InitialCondition=controlDeflections(2)
  Saturation : Saturate  UpperLimit=20  LowerLimit=-20
  Saturation1 : Saturate  UpperLimit=60  LowerLimit=-60
  Sum1 : Sum  Inputs=|+-
  Output : Outport
  wires:
  Saturation1/1 -> Integrator/1
  Gain/1 -> Saturation1/1
  Sum1/1 -> Gain/1
  Deflection/1 -> Sum1/1
  Integrator/1 -> Saturation/1
  Saturation/1 -> Output/1, Sum1/2
  [Reset] -> Integrator/2

== system F16_Quaternion/Actuator Module/First Order HT Actuator ==
  Deflection : Inport
  Gain : Gain  Gain=1/0.0495
  Integrator : Integrator  ExternalReset=either  InitialCondition=controlDeflections(1)
  Saturation : Saturate  UpperLimit=25  LowerLimit=-25
  Saturation1 : Saturate  UpperLimit=60  LowerLimit=-60
  Sum1 : Sum  Inputs=|+-
  Output : Outport
  wires:
  Sum1/1 -> Gain/1
  Gain/1 -> Saturation1/1
  Integrator/1 -> Saturation/1
  Saturation1/1 -> Integrator/1
  Deflection/1 -> Sum1/1
  Saturation/1 -> Output/1, Sum1/2
  [Reset] -> Integrator/2

== system F16_Quaternion/Actuator Module/First Order Rudder Actuator ==
  Deflection : Inport
  Gain : Gain  Gain=1/0.0495
  Integrator : Integrator  ExternalReset=either  InitialCondition=controlDeflections(3)
  Saturation : Saturate  UpperLimit=30  LowerLimit=-30
  Saturation1 : Saturate  UpperLimit=120  LowerLimit=-120
  Sum1 : Sum  Inputs=|+-
  Output : Outport
  wires:
  Sum1/1 -> Gain/1
  Gain/1 -> Saturation1/1
  Saturation/1 -> Output/1, Sum1/2
  Saturation1/1 -> Integrator/1
  Deflection/1 -> Sum1/1
  Integrator/1 -> Saturation/1
  [Reset] -> Integrator/2

== system F16_Quaternion/Actuator Module/First Order Throttle Actuator ==
  Deflection : Inport
  Gain : Gain  Gain=1/0.0495
  Integrator : Integrator  ExternalReset=either  InitialCondition=controlDeflections(4)
  Saturation : Saturate  UpperLimit=100  LowerLimit=0
  Saturation1 : Saturate  UpperLimit=30  LowerLimit=-30
  Sum1 : Sum  Inputs=|+-
  Output : Outport
  wires:
  [Reset] -> Integrator/2
  Integrator/1 -> Saturation/1
  Deflection/1 -> Sum1/1
  Saturation1/1 -> Integrator/1
  Saturation/1 -> Sum1/2, Output/1
  Gain/1 -> Saturation1/1
  Sum1/1 -> Gain/1

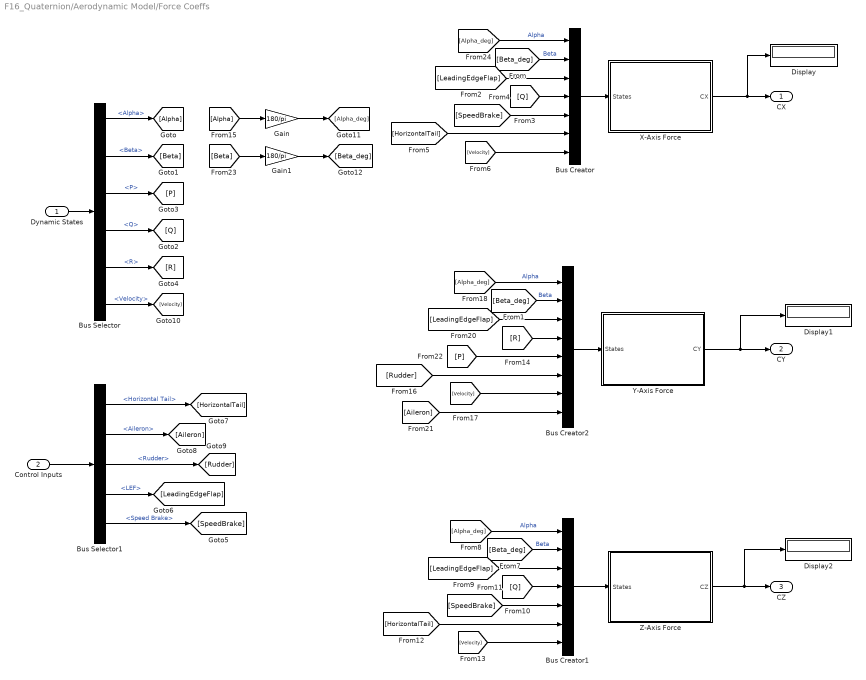
== system F16_Quaternion/Aerodynamic Model/Force Coeffs ==
  Dynamic States : Inport
  Control Inputs : Inport  Port=2
  Bus Creator : BusCreator  Inputs=7
  Bus Creator1 : BusCreator  Inputs=7
  Bus Creator2 : BusCreator  Inputs=8
  Bus Selector : BusSelector  OutputSignals=Alpha,Beta,P,Q,R,Velocity
  Bus Selector1 : BusSelector  OutputSignals=Horizontal Tail,Aileron,Rudder,LEF,Speed Brake
  Display : Display
  Display1 : Display
  Display2 : Display
  Gain : Gain  Gain=180/pi
  Gain1 : Gain  Gain=180/pi
  X-Axis Force : Subsystem
  Y-Axis Force : Subsystem
  Z-Axis Force : Subsystem
  " CX" : Outport  VectorParamsAs1DForOutWhenUnconnected=off
  " CY" : Outport  Port=2  VectorParamsAs1DForOutWhenUnconnected=off
  " CZ" : Outport  Port=3  VectorParamsAs1DForOutWhenUnconnected=off
  wires:
  Dynamic States/1 -> Bus Selector/1
  Bus Creator/1 -> X-Axis Force/1(States)
  X-Axis Force/1(CX) -> Display/1, " CX"/1
  Y-Axis Force/1(CY) -> Display1/1, " CY"/1
  Z-Axis Force/1(CZ) -> Display2/1, " CZ"/1
  [Alpha_deg] -> Bus Creator/1  "Alpha"
  [Beta_deg] -> Bus Creator/2  "Beta"
  [LeadingEdgeFlap] -> Bus Creator/3
  [Q] -> Bus Creator/4
  [SpeedBrake] -> Bus Creator/5
  [HorizontalTail] -> Bus Creator/6
  [Velocity] -> Bus Creator/7
  [Velocity] -> Bus Creator1/7
  [HorizontalTail] -> Bus Creator1/6
  [SpeedBrake] -> Bus Creator1/5
  [Q] -> Bus Creator1/4
  [LeadingEdgeFlap] -> Bus Creator1/3
  Bus Creator1/1 -> Z-Axis Force/1(States)
  [LeadingEdgeFlap] -> Bus Creator2/3
  [R] -> Bus Creator2/4
  [Rudder] -> Bus Creator2/6
  [Velocity] -> Bus Creator2/7
  Bus Creator2/1 -> Y-Axis Force/1(States)
  [Aileron] -> Bus Creator2/8
  [P] -> Bus Creator2/5
  Bus Selector/1 -> [Alpha]  "<Alpha>"
  Bus Selector/2 -> [Beta]  "<Beta>"
  Bus Selector/3 -> [P]  "<P>"
  Bus Selector/4 -> [Q]  "<Q>"
  Bus Selector/5 -> [R]  "<R>"
  Bus Selector/6 -> [Velocity]  "<Velocity>"
  Control Inputs/1 -> Bus Selector1/1
  Bus Selector1/1 -> [HorizontalTail]  "<Horizontal Tail>"
  Bus Selector1/2 -> [Aileron]  "<Aileron>"
  Bus Selector1/3 -> [Rudder]  "<Rudder>"
  Bus Selector1/4 -> [LeadingEdgeFlap]  "<LEF>"
  Bus Selector1/5 -> [SpeedBrake]  "<Speed Brake>"
  [Alpha] -> Gain/1
  Gain/1 -> [Alpha_deg]
  [Beta] -> Gain1/1
  Gain1/1 -> [Beta_deg]
  [Alpha_deg] -> Bus Creator2/1  "Alpha"
  [Beta_deg] -> Bus Creator2/2  "Beta"
  [Alpha_deg] -> Bus Creator1/1  "Alpha"
  [Beta_deg] -> Bus Creator1/2  "Beta"

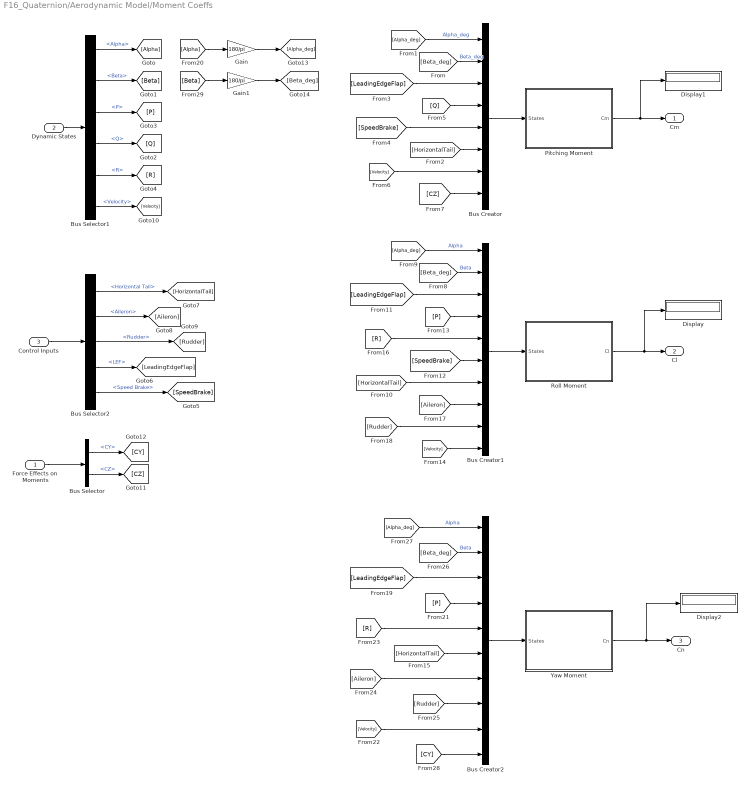
== system F16_Quaternion/Aerodynamic Model/Moment Coeffs ==
  Force Effects on Moments : Inport
  Dynamic States : Inport  Port=2
  Control Inputs : Inport  Port=3
  Bus Creator : BusCreator  Inputs=8
  Bus Creator1 : BusCreator  Inputs=10
  Bus Creator2 : BusCreator  Inputs=10
  Bus Selector : BusSelector  OutputSignals=CY,CZ
  Bus Selector1 : BusSelector  OutputSignals=Alpha,Beta,P,Q,R,Velocity
  Bus Selector2 : BusSelector  OutputSignals=Horizontal Tail,Aileron,Rudder,LEF,Speed Brake
  Display : Display
  Display1 : Display
  Display2 : Display
  Gain : Gain  Gain=180/pi
  Gain1 : Gain  Gain=180/pi
  Pitching Moment : Subsystem
  Roll Moment : Subsystem
  Yaw Moment : Subsystem
  " Cm" : Outport
  " Cl" : Outport  Port=2
  " Cn" : Outport  Port=3
  wires:
  Pitching Moment/1(Cm) -> Display1/1, " Cm"/1
  Bus Creator/1 -> Pitching Moment/1(States)
  [SpeedBrake] -> Bus Creator/5
  [LeadingEdgeFlap] -> Bus Creator/3
  [Q] -> Bus Creator/4
  [HorizontalTail] -> Bus Creator/6
  [Velocity] -> Bus Creator/7
  [CZ] -> Bus Creator/8
  Force Effects on Moments/1 -> Bus Selector/1
  Bus Selector/1 -> [CY]  "<CY>"
  Bus Selector/2 -> [CZ]  "<CZ>"
  [P] -> Bus Creator1/4
  [LeadingEdgeFlap] -> Bus Creator1/3
  Roll Moment/1(Cl) -> Display/1, " Cl"/1
  Yaw Moment/1(Cn) -> Display2/1, " Cn"/1
  [Velocity] -> Bus Creator1/10
  [R] -> Bus Creator1/5
  [SpeedBrake] -> Bus Creator1/6
  [HorizontalTail] -> Bus Creator1/7
  [Aileron] -> Bus Creator1/8
  [Rudder] -> Bus Creator1/9
  [Rudder] -> Bus Creator2/8
  [Aileron] -> Bus Creator2/7
  [HorizontalTail] -> Bus Creator2/6
  [R] -> Bus Creator2/5
  [Velocity] -> Bus Creator2/9
  [LeadingEdgeFlap] -> Bus Creator2/3
  [P] -> Bus Creator2/4
  Bus Creator2/1 -> Yaw Moment/1(States)
  Bus Selector1/4 -> [Q]  "<Q>"
  Bus Selector2/1 -> [HorizontalTail]  "<Horizontal Tail>"
  Control Inputs/1 -> Bus Selector2/1
  Bus Selector2/5 -> [SpeedBrake]  "<Speed Brake>"
  Bus Selector2/2 -> [Aileron]  "<Aileron>"
  Bus Selector1/6 -> [Velocity]  "<Velocity>"
  Bus Selector1/3 -> [P]  "<P>"
  Bus Selector1/2 -> [Beta]  "<Beta>"
  Bus Selector2/3 -> [Rudder]  "<Rudder>"
  Bus Selector1/5 -> [R]  "<R>"
  Bus Selector2/4 -> [LeadingEdgeFlap]  "<LEF>"
  Dynamic States/1 -> Bus Selector1/1
  Bus Selector1/1 -> [Alpha]  "<Alpha>"
  Bus Creator1/1 -> Roll Moment/1(States)
  Gain1/1 -> [Beta_deg]
  [Beta] -> Gain1/1
  [Alpha] -> Gain/1
  Gain/1 -> [Alpha_deg]
  [Alpha_deg] -> Bus Creator/1  "Alpha_deg"
  [Beta_deg] -> Bus Creator/2  "Beta_deg"
  [Alpha_deg] -> Bus Creator1/1  "Alpha"
  [Beta_deg] -> Bus Creator1/2  "Beta"
  [Alpha_deg] -> Bus Creator2/1  "Alpha"
  [Beta_deg] -> Bus Creator2/2  "Beta"
  [CY] -> Bus Creator2/10

== system F16_Quaternion/Equations of Motion (Quat)/Acisal_Ivme_Hesaplari ==
  note: Açısal İvme Hesapları
  note: ÇIKTILAR
  note: GİRDİLER
  p q r : Inport  OutDataTypeStr=double
  I : Inport  Port=2  OutDataTypeStr=double
  Moments : Inport  Port=3  OutDataTypeStr=double
  Add : Sum  Inputs=+-
  Cross Product : matrix_library/Cross Product
  Product2 : Product  Inputs=*/  Multiplication=Matrix(*)  SaturateOnIntegerOverflow=on  OutDataTypeStr=Inherit: Same as first input
  Reshape : Reshape
  Reshape1 : Reshape  OutputDimensionality=Row vector (2-D)
  Subsystem : Subsystem
  pdot qdot rdot : Outport  OutDataTypeStr=double  VectorParamsAs1DForOutWhenUnconnected=off
  wires:
  I/1 -> [I]
  Moments/1 -> [Moments]
  p q r/1 -> [p_q_r_rad_sn]
  [I] -> Product2/2
  [Moments] -> Add/1
  [I] -> Subsystem/2(Inertia)
  Reshape1/1 -> Product2/1
  Reshape/1 -> pdot qdot rdot/1
  Product2/1 -> Reshape/1
  Cross Product/1 -> Add/2
  [p_q_r_rad_sn] -> Cross Product/1, Subsystem/1(p q r)
  Subsystem/1(I * w) -> Cross Product/2
  Add/1 -> Reshape1/1

== system F16_Quaternion/Equations of Motion (Quat)/Subsystem ==
  x_y_z_m : Outport  OutDataTypeStr=double  Unit=m  VectorParamsAs1DForOutWhenUnconnected=off
  Dusey_Hiz_m_sn : Outport  Port=2  OutDataTypeStr=double  Unit=m/s  VectorParamsAs1DForOutWhenUnconnected=off
  Yatay_Hiz_m_sn : Outport  Port=3  OutDataTypeStr=double  Unit=m/s  VectorParamsAs1DForOutWhenUnconnected=off
  u_v_w_m_sn : Outport  Port=4  OutDataTypeStr=double  Unit=m/s  VectorParamsAs1DForOutWhenUnconnected=off
  dot_u_v_w_m_sn : Outport  Port=5  OutDataTypeStr=double  Unit=m/s^2  VectorParamsAs1DForOutWhenUnconnected=off
  phi_theta_psi_rad : Outport  Port=6  OutDataTypeStr=double  Unit=rad  VectorParamsAs1DForOutWhenUnconnected=off
  p,q,r : Outport  Port=7  OutDataTypeStr=double  Unit=rad/s  VectorParamsAs1DForOutWhenUnconnected=off
  dot_p_q_r_rad_sn : Outport  Port=8  OutDataTypeStr=double  Unit=rad/s^2  VectorParamsAs1DForOutWhenUnconnected=off
  DCM_b2e : Outport  Port=9  OutDataTypeStr=double  Unit=1  VectorParamsAs1DForOutWhenUnconnected=off

== system F16_Quaternion/Equations of Motion (Quat)/dot_quat ==
  p q r : Inport
  q0 q1 q2 q3 : Inport  Port=2
  Constant : Constant
  Dot Product : DotProduct  InputSameDT=off  OutDataTypeStr=Inherit: Inherit via internal rule
  High Gain Quaternion Normalization : Gain  SaturateOnIntegerOverflow=on  OutDataTypeStr=Inherit: Same as input  ParamDataTypeStr=Inherit: Same as input
  Mux1 : Mux  Inputs=[3 4 1]
  Mux2 : Mux
  Sum : Sum  Inputs=|+-  InputSameDT=on  SaturateOnIntegerOverflow=on  OutDataTypeStr=Inherit: Same as first input
  q0dot : Fcn  Expr=-0.5 * ( u[5]*u[1]+u[6]*u[2]+u[7]*u[3] ) + u[8]*u[4]
  q1dot : Fcn  Expr=0.5 * ( u[4]*u[1]+u[6]*u[3]-u[7]*u[2] ) + u[8]*u[5]
  q2dot : Fcn  Expr=0.5 * ( u[4]*u[2]+u[7]*u[1]-u[5]*u[3] ) + u[8]*u[6]
  q3dot : Fcn  Expr=0.5 * ( u[4]*u[3]+u[5]*u[2]-u[6]*u[1] ) + u[8]*u[7]
  qdot : Outport  InitialOutput=0  VectorParamsAs1DForOutWhenUnconnected=off
  wires:
  q0dot/1 -> Mux2/1
  q3dot/1 -> Mux2/4
  q0 q1 q2 q3/1 -> Mux1/2, Dot Product/2, Dot Product/1
  Sum/1 -> High Gain Quaternion Normalization/1
  Mux2/1 -> qdot/1
  q1dot/1 -> Mux2/2
  Constant/1 -> Sum/1
  q2dot/1 -> Mux2/3
  High Gain Quaternion Normalization/1 -> Mux1/3
  Mux1/1 -> q1dot/1, q0dot/1, q3dot/1, q2dot/1
  p q r/1 -> Mux1/1
  Dot Product/1 -> Sum/2

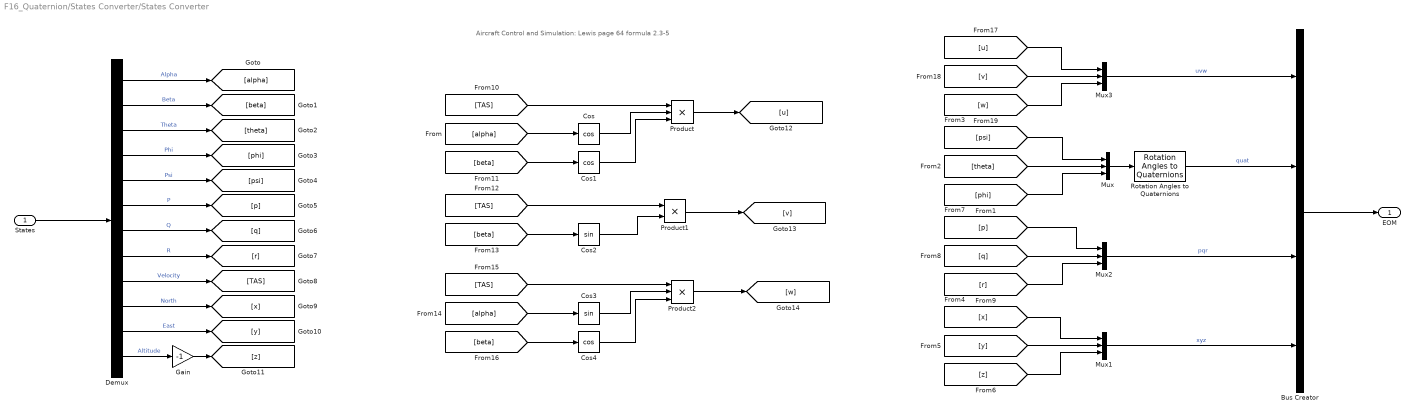
== system F16_Quaternion/States Converter/States Converter ==
  note: Aircraft Control and Simulation: Lewis page 64 formula 2.3-5
  States : Inport
  Bus Creator : BusCreator  Inputs=4
  Cos : Trigonometry  Operator=cos
  Cos1 : Trigonometry  Operator=cos
  Cos2 : Trigonometry
  Cos3 : Trigonometry
  Cos4 : Trigonometry  Operator=cos
  Demux : Demux  Outputs=12
  Gain : Gain  Gain=-1
  Mux{,1..3} (4 alike) : Mux  Inputs=3
  Product : Product  Inputs=***
  Product1 : Product  Inputs=**
  Product2 : Product  Inputs=***
  Rotation Angles to Quaternions : sharedtransform/Rotation Angles to Quaternions  rotationOrder=ZYX  aMode=aMode
  EOM : Outport
  wires:
  [w] -> Mux3/3
  [u] -> Mux3/1
  [v] -> Mux3/2
  Product2/1 -> [w]
  [alpha] -> Cos3/1
  [beta] -> Cos4/1
  Cos3/1 -> Product2/2
  Cos4/1 -> Product2/3
  [TAS] -> Product2/1
  Product1/1 -> [v]
  Product/1 -> [u]
  [TAS] -> Product1/1
  Cos2/1 -> Product1/2
  [beta] -> Cos2/1
  [TAS] -> Product/1
  Cos1/1 -> Product/3
  Cos/1 -> Product/2
  [beta] -> Cos1/1
  [alpha] -> Cos/1
  [p] -> Mux2/1
  [r] -> Mux2/3
  [q] -> Mux2/2
  [z] -> Mux1/3
  [x] -> Mux1/1
  [y] -> Mux1/2
  Mux1/1 -> Bus Creator/4  "xyz"
  Bus Creator/1 -> EOM/1
  Mux2/1 -> Bus Creator/3  "pqr"
  Mux3/1 -> Bus Creator/1  "uvw"
  [phi] -> Mux/3
  [psi] -> Mux/1
  [theta] -> Mux/2
  Mux/1 -> Rotation Angles to Quaternions/1
  Rotation Angles to Quaternions/1 -> Bus Creator/2  "quat"
  Gain/1 -> [z]
  Demux/12 -> Gain/1  "Altitude"
  Demux/11 -> [y]  "East"
  Demux/10 -> [x]  "North"
  Demux/9 -> [TAS]  "Velocity"
  Demux/8 -> [r]  "R"
  Demux/7 -> [q]  "Q"
  Demux/6 -> [p]  "P"
  Demux/5 -> [psi]  "Psi"
  Demux/4 -> [phi]  "Phi"
  Demux/3 -> [theta]  "Theta"
  Demux/2 -> [beta]  "Beta"
  Demux/1 -> [alpha]  "Alpha"
  States/1 -> Demux/1

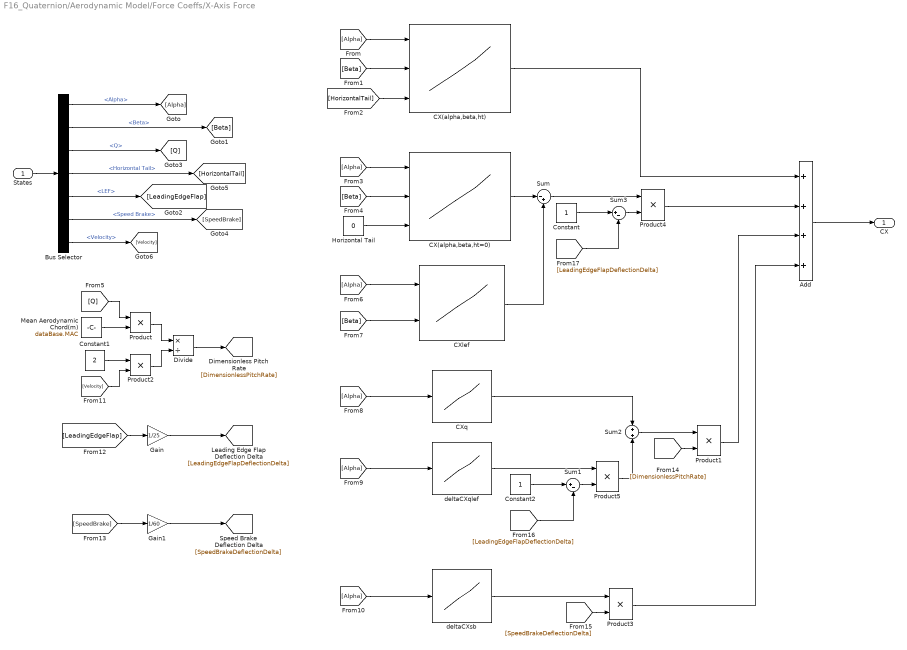
== system F16_Quaternion/Aerodynamic Model/Force Coeffs/X-Axis Force ==
  States : Inport
  Add : Sum  Inputs=++++
  Bus Selector : BusSelector  OutputSignals=Alpha,Beta,Q,Horizontal Tail,LEF,Speed Brake,Velocity
  CX(alpha,beta,ht) : Lookup_n-D  NumberOfTableDimensions=3  BreakpointsForDimension1=dataBase.f16_AerodynamicData.BP.CX.CX.alpha  BreakpointsForDimension2=dataBase.f16_AerodynamicData.BP.CX.CX.beta  BreakpointsForDimension3=dataBase.f16_AerodynamicData.BP.CX.CX.dHT  Table=dataBase.f16_AerodynamicData.data.CX.CX  InternalRulePriority=Speed  RndMeth=Simplest
      settings: InputPortMap=u0,u1,u2
  CX(alpha,beta,ht=0) : Lookup_n-D  NumberOfTableDimensions=3  BreakpointsForDimension1=dataBase.f16_AerodynamicData.BP.CX.CX.alpha  BreakpointsForDimension2=dataBase.f16_AerodynamicData.BP.CX.CX.beta  BreakpointsForDimension3=dataBase.f16_AerodynamicData.BP.CX.CX.dHT  Table=dataBase.f16_AerodynamicData.data.CX.CX  InternalRulePriority=Speed  RndMeth=Simplest
      settings: InputPortMap=u0,u1,u2
  CXlef : Lookup_n-D  BreakpointsForDimension1=dataBase.f16_AerodynamicData.BP.CX.CXlef.alpha  BreakpointsForDimension2=dataBase.f16_AerodynamicData.BP.CX.CXlef.beta  Table=dataBase.f16_AerodynamicData.data.CX.CXlef  InternalRulePriority=Speed  RndMeth=Simplest
      settings: InputPortMap=u0,u1
  CXq : Lookup_n-D  NumberOfTableDimensions=1  BreakpointsForDimension1=dataBase.f16_AerodynamicData.BP.CX.CXq.alpha  Table=dataBase.f16_AerodynamicData.data.CX.CXq  InternalRulePriority=Speed  RndMeth=Simplest
  Constant : Constant
  Constant1 : Constant  Value=2
  Constant2 : Constant
  Divide : Product  Inputs=*/
  Gain : Gain  Gain=1/25
  Gain1 : Gain  Gain=1/60
  Horizontal Tail : Constant  Value=0
  Mean Aerodynamic Chord(m) : Constant  Value=dataBase.MAC
  Product{,1..5} (6 alike) : Product
  Sum : Sum  Inputs=|-+
  Sum1 : Sum  Inputs=|+-
  Sum2 : Sum  Inputs=+|+
  Sum3 : Sum  Inputs=|+-
  deltaCXqlef : Lookup_n-D  NumberOfTableDimensions=1  BreakpointsForDimension1=dataBase.f16_AerodynamicData.BP.CX.deltaCXqlef.alpha  Table=dataBase.f16_AerodynamicData.data.CX.deltaCXqlef  InternalRulePriority=Speed  RndMeth=Simplest
  deltaCXsb : Lookup_n-D  NumberOfTableDimensions=1  BreakpointsForDimension1=dataBase.f16_AerodynamicData.BP.CX.deltaCXSB.alpha  Table=dataBase.f16_AerodynamicData.data.CX.deltaCXSB  InternalRulePriority=Speed  RndMeth=Simplest
  CX : Outport  VectorParamsAs1DForOutWhenUnconnected=off
  wires:
  States/1 -> Bus Selector/1
  [Alpha] -> CX(alpha,beta,ht)/1
  [Beta] -> CX(alpha,beta,ht)/2
  [HorizontalTail] -> CX(alpha,beta,ht)/3
  [Alpha] -> CX(alpha,beta,ht=0)/1
  Horizontal Tail/1 -> CX(alpha,beta,ht=0)/3
  [Beta] -> CX(alpha,beta,ht=0)/2
  CX(alpha,beta,ht=0)/1 -> Sum/1
  CXlef/1 -> Sum/2
  [Alpha] -> CXlef/1
  [Beta] -> CXlef/2
  [Alpha] -> CXq/1
  [Alpha] -> deltaCXqlef/1
  [Alpha] -> deltaCXsb/1
  [Q] -> Product/1
  Mean Aerodynamic Chord(m)/1 -> Product/2
  Product/1 -> Divide/1
  Divide/1 -> [DimensionlessPitchRate]
  Add/1 -> CX/1
  CX(alpha,beta,ht)/1 -> Add/1
  [LeadingEdgeFlap] -> Gain/1
  [SpeedBrake] -> Gain1/1
  Gain1/1 -> [SpeedBrakeDeflectionDelta]
  CXq/1 -> Sum2/1
  Sum2/1 -> Product1/1
  Constant1/1 -> Product2/1
  [Velocity] -> Product2/2
  Product2/1 -> Divide/2
  [DimensionlessPitchRate] -> Product1/2
  deltaCXsb/1 -> Product3/1
  [SpeedBrakeDeflectionDelta] -> Product3/2
  Product1/1 -> Add/3
  Product3/1 -> Add/4
  Sum/1 -> Product4/1
  Product4/1 -> Add/2
  Gain/1 -> [LeadingEdgeFlapDeflectionDelta]
  Constant/1 -> Sum3/1
  Sum3/1 -> Product4/2
  [LeadingEdgeFlapDeflectionDelta] -> Sum3/2
  [LeadingEdgeFlapDeflectionDelta] -> Sum1/2
  Constant2/1 -> Sum1/1
  Product5/1 -> Sum2/2
  deltaCXqlef/1 -> Product5/1
  Sum1/1 -> Product5/2
  Bus Selector/1 -> [Alpha]  "<Alpha>"
  Bus Selector/2 -> [Beta]  "<Beta>"
  Bus Selector/3 -> [Q]  "<Q>"
  Bus Selector/4 -> [HorizontalTail]  "<Horizontal Tail>"
  Bus Selector/5 -> [LeadingEdgeFlap]  "<LEF>"
  Bus Selector/6 -> [SpeedBrake]  "<Speed Brake>"
  Bus Selector/7 -> [Velocity]  "<Velocity>"
